simulink model "test_reg"  (Simulink 7.6)
settings: Solver=ode4  StartTime=0.0  StopTime=10.0  FixedStep=0.001  RelTol=1e-3
settings Model: Creator=jordan  LastModifiedBy=jordan

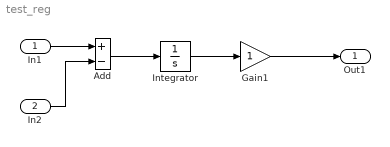
== system test_reg ==
  In1 : Inport
  In2 : Inport  Port=2
  Add : Sum  Inputs=+-
  Gain1 : Gain
  Integrator : Integrator
  Out1 : Outport
  wires:
  Add/1 -> Integrator/1
  Integrator/1 -> Gain1/1
  In1/1 -> Add/1
  In2/1 -> Add/2
  Gain1/1 -> Out1/1
